simulink model "LAB6"  (R2025b)
settings: Solver=VariableStepAuto  StartTime=0.0  StopTime=100  RelTol=1e-3
settings Model: Creator=Wingshingsho  LastModifiedBy=Wingshingsho

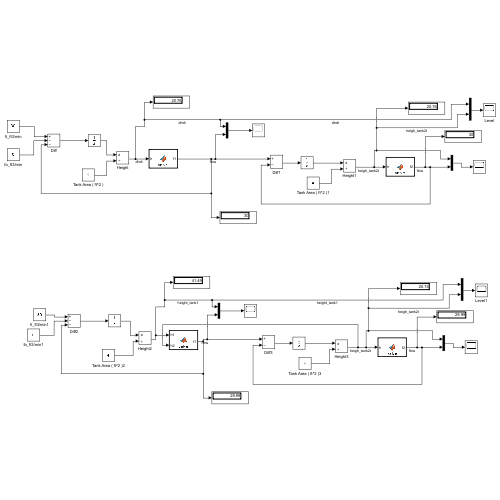
[thumbnail: Simulink's stored preview of the top-level diagram]
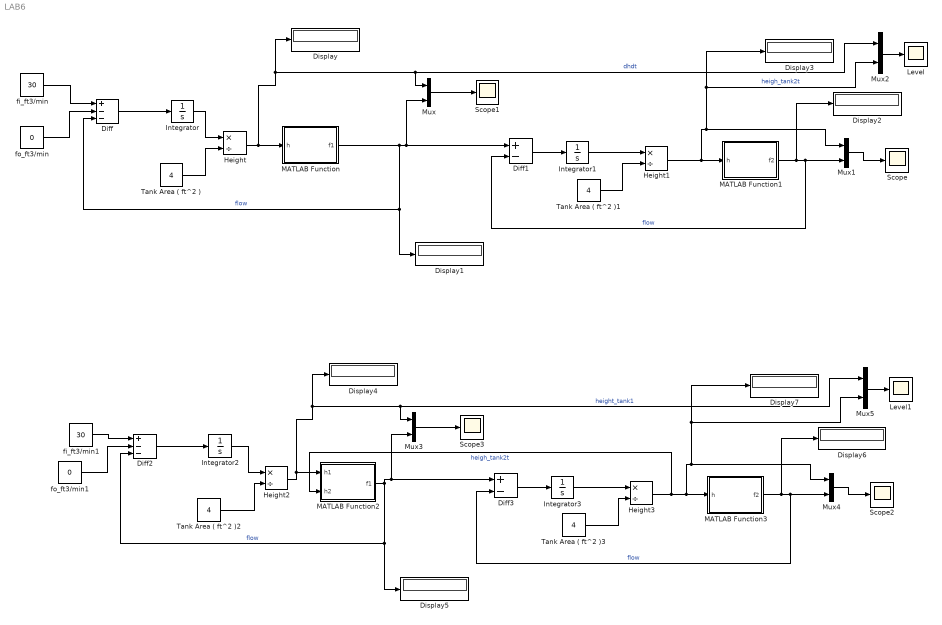
== system LAB6 ==
  Diff : Sum  Inputs=+--
  Diff1 : Sum  Inputs=+-
  Diff2 : Sum  Inputs=+--
  Diff3 : Sum  Inputs=+-
  Display{,1..7} (8 alike) : Display
  Height{,1..3} (4 alike) : Product  Inputs=*/
  Integrator{,1..3} (4 alike) : Integrator
  Level : Scope
      settings: ActiveDisplayYMinimum=-2.5951156687586296  ActiveDisplayYMaximum=23.356041018827671  DataLoggingVariableName=ScopeData2
  Level1 : Scope
      settings: ActiveDisplayYMinimum=-5.1866326305686812  ActiveDisplayYMaximum=46.679693675118138  DataLoggingVariableName=ScopeData3
  MATLAB Function : MATLAB Function  TreatAsAtomicUnit=on
  MATLAB Function1 : MATLAB Function  TreatAsAtomicUnit=on
  MATLAB Function2 : MATLAB Function  TreatAsAtomicUnit=on
  MATLAB Function3 : MATLAB Function  TreatAsAtomicUnit=on
  Mux{,1..5} (6 alike) : Mux  Inputs=2
  Scope{,1..3} (4 alike) : Scope
      Scope settings: ActiveDisplayYMinimum=-1  ActiveDisplayYMaximum=1
      Scope1 settings: ActiveDisplayYMinimum=-3.7499999802666588  ActiveDisplayYMaximum=33.749999822399936
      Scope2 settings: ActiveDisplayYMinimum=-1  ActiveDisplayYMaximum=1  DataLoggingVariableName=ScopeData4
      Scope3 settings: ActiveDisplayYMinimum=-3.7438754161647805  ActiveDisplayYMaximum=33.694878745483031  DataLoggingVariableName=ScopeData5
  Tank Area ( ft^2 ){,1..3} (4 alike) : Constant  Value=4
  fi_ft3/min : Constant  Value=30
  fi_ft3/min1 : Constant  Value=30
  fo_ft3/min : Constant  Value=0
  fo_ft3/min1 : Constant  Value=0
  wires:
  fi_ft3/min/1 -> Diff/1
  fo_ft3/min/1 -> Diff/2
  Diff/1 -> Integrator/1
  Integrator/1 -> Height/1
  Tank Area ( ft^2 )/1 -> Height/2
  Height/1 -> Display/1, Mux2/1, Mux/1, MATLAB Function/1(h)  "dhdt"
  MATLAB Function/1(f1) -> Diff/3, Display1/1, Diff1/1, Mux/2  "flow"
  Diff1/1 -> Integrator1/1
  Integrator1/1 -> Height1/1
  Tank Area ( ft^2 )1/1 -> Height1/2
  Height1/1 -> Mux2/2, Display3/1, Mux1/1, MATLAB Function1/1(h)  "heigh_tank2t"
  MATLAB Function1/1(f2) -> Display2/1, Mux1/2, Diff1/2  "flow"
  Mux/1 -> Scope1/1
  Mux1/1 -> Scope/1
  Mux2/1 -> Level/1
  Mux4/1 -> Scope2/1
  Height3/1 -> MATLAB Function2/2(h2), Mux5/2, Display7/1, Mux4/1, MATLAB Function3/1(h)  "heigh_tank2t"
  Mux3/1 -> Scope3/1
  MATLAB Function3/1(f2) -> Display6/1, Mux4/2, Diff3/2  "flow"
  Tank Area ( ft^2 )3/1 -> Height3/2
  Mux5/1 -> Level1/1
  MATLAB Function2/1(f1) -> Diff3/1, Mux3/2, Diff2/3, Display5/1  "flow"
  Height2/1 -> Display4/1, Mux5/1, Mux3/1, MATLAB Function2/1(h1)  "height_tank1"
  Integrator3/1 -> Height3/1
  Diff3/1 -> Integrator3/1
  Diff2/1 -> Integrator2/1
  fo_ft3/min1/1 -> Diff2/2
  fi_ft3/min1/1 -> Diff2/1
  Integrator2/1 -> Height2/1
  Tank Area ( ft^2 )2/1 -> Height2/2

== matlab function LAB6/MATLAB Function ==
  data: h input; f1 output
function f1 = valve(h)
Cv = 75 * 0.13336;
LHO = 70;
SG = LHO / 62.4;
Pressure = ( LHO * h )/144;
f1 = Cv * (SG)^-0.5 * ((Pressure)^0.5);

end

== matlab function LAB6/MATLAB Function2 ==
  data: h1 input; f1 output; h2 input
function f1 = valve(h1,h2)
Cv = 75 * 0.13336;
LHO = 70;
SG = LHO / 62.4;
Pressure = ( LHO * (h1-h2) )/144;
if Pressure > 0
    f1 = Cv * (SG)^-0.5 * ((Pressure)^0.5);
else
    f1 = 0;
end

end

== matlab function LAB6/MATLAB Function3 ==
  data: h input; f2 output
function f2 = valve(h)
Cv = 75 * 0.13336;
LHO = 70;
SG = LHO / 62.4;
Pressure = ( LHO * h )/144;
f2 = Cv * (SG)^-0.5 * ((Pressure)^0.5);

end

== matlab function LAB6/MATLAB Function1 ==
  data: h input; f2 output
function f2 = valve(h)
Cv = 75 * 0.13336;
LHO = 70;
SG = LHO / 62.4;
Pressure = ( LHO * h )/144;
f2 = Cv * (SG)^-0.5 * ((Pressure)^0.5);

end
